simulink library "SUB_ECU_L4_MABX_HW_Interface_PIC_PB"  (R2018a)
settings: Solver=VariableStepAuto  StartTime=0.0  StopTime=10.0  RelTol=1e-3
PostLoadFcn:
  | , if any(exist('dsrtsu_mdlpostloadfcn', 'file') == [2, 3, 6]), try dsrtsu_mdlpostloadfcn('Execute', bdroot); catch fprintf('Error in PostLoadFcn (dsrtsu_mdlpostloadfcn) for model "%s":\n %s\n', bdroot, lasterr); end, end,
undefined symbols (not defined in the file or in its folder): CANR_PROPB_REAX_3_13_CHANNEL_APV, CANR_PROPB_REAX_4_13_CHANNEL_APV, CANR_PROPB_XPR_1_50_CHANNEL_APV, ENUM_CAN_RX_T, ENUM_CAN_TX_T, ENUM_REAX_OPERATION_MODE_T, ENUM_SIGNAL_HEALTH_T, ENUM_XBR_CONTROL_MODE_T, ENUM_XBR_EBI_MODE_T, ENUM_XBR_PASS_THROUGH_ACTIVE_T, ENUM_XBR_PRIORITY_T, ENUM_XPR_INHIBIT_PARK_MANUAL_T, ENUM_XPR_INHIBIT_UNPARK_MANUAL_T, ENUM_XPR_PARK_MANUAL_T, ENUM_XPR_UNPARK_MANUAL_T, PROPB_REAX_1_E4_DES_POS_SIG_SRC_APV, PROPB_REAX_1_E4_DESIRED_OPMODE_APV, PROPB_REAX_1_E4_DESIRED_POSITION_APV, PROPB_REAX_CHANNEL_APV, ptc_matlab_lib
libraries: PTC_MBDS_LIB x293, rtican x158, simulink x61, EmE_MBD_Blockset x38, rti1401lib_dio_type4 x14, simulink_need_slupdate x7, $bdroot x5, rti1401lib_adc_type4 x3, rtmapslib x3, dsa_tcpip_lib x2, SUB_ECU_L4_MABX_HW_Interface_PTC_1571 x1, rtitasklib x1
(part 3 of 49)

== system SUB_ECU_L4_MABX_HW_Interface_PIC_PB/DIGITAL ==
  ADC_TYPE4_BL1 : rti1401lib_adc_type4/ADC_TYPE4_BL1  DSProperties=struct('RTI',struct('Version',uint32(2),'BlockType',struct('isSLSource',uint8(1),'isSLSink',uint8(1),'isHWSource',uint8(0),'isHWSink',uint8(1),'isSetup',uint8(0),'isInline',uint8(1),'isNonInline',uint8(0),'isInterrupt',uint8(0),'isChannelwise',uint8(1)),'IOBoardType',{{'DS1401','STD','ADCT4'}},'UnitType','ADC','Identifier','ADC','DialogType','ML','BlockSet','NONE','SlaveProcessor','NONE'))  RTIBlockInterface=struct('InputPortsActive',0,'InputPortsWidth',int32(1),'InputPortsDataType',{{'SS_BOOLEAN'}},'InputPortsName',{{'Continue'}},'OutputPortsActive',[1 0],'OutputPortsWidth',int32([1 1]),'OutputPortsDataType',{{'SS_DOUBLE','SS_UINT8'}},'OutputPortsName',{{'ADC','Status'}},'DialogFcn','rti1401stdadct4adcgui','SampleTime',{{-1}},'InitLevel',3,'IconTransparency','on','BlockDisplay',{{['ADC TP4\nModule: 1\nChannel: 2'],'center'}},'BlockName',struct('Token',{{'ADC_TYPE4_BL1'}}))  RTIBlockParameters=struct('ADCSWStartDisable',{{0,'OFF',[0 1]}},'ModuleNo',{{1,'OFF',[1 16]}},'ChannelNo',{{2,'OFF',[1 16]}},'ConversionMode',{{1,'OFF',[1 2]}},'SampleMode',{{1,'OFF',[1 2]}},'TriggerSource',{{1,'OFF',[1 5]}},'EdgePolarity',{{1,'OFF',[1 2]}},'ConversionTriggerSource',{{2,'OFF',[1 6]}},'ConversionEdgePolarity',{{1,'OFF',[1 2]}},'ConversionPeriod',{{'1e-06','OFF',[]}},'ConversionPeriodCheck',{{0,'OFF',[]}},'BurstTriggerSource',{{1,'OFF',[1 6]}},'BurstEdgePolarity',{{1,'OFF',[1 2]}},'BurstSize',{{'10','OFF',[]}},'BurstSizeCheck',{{0,'OFF',[]}},'DataSetOffset',{{'0','OFF',[]}},'DataSetOffsetCheck',{{0,'OFF',[]}},'DataSetLength',{{'1','OFF',[]}},'DataSetLengthCheck',{{0,'OFF',[]}},'ReadMode',{{1,'OFF',[1 2]}},'SampleTime',{{'-1','OFF',[-1 inf]}},'SampleTimeCheck',{{1,'OFF',[]}},'StatusPortEnable',{{0,'OFF',[0 1]}},'VoltageRange',{{2,'OFF',[1 2]}},'TLCFileName',{{'rti1401adc_t4_adc','OFF',[]}})  RTISFcnParameters=struct('ADCSWStartDisable','int32','ModuleNo','int32','ChannelNo','int16','ConversionMode','int16','SampleMode','int16','TriggerSource','int16','EdgePolarity','int16','ConversionTriggerSource','int16','ConversionEdgePolarity','int16','ConversionPeriod','double','BurstTriggerSource','int16','BurstEdgePolarity','int16','BurstSize','int16','DataSetOffset','int16','DataSetLength','int16','ReadMode','int16','SampleTime','double','StatusPortEnable','int16','VoltageRange','int16','TLCFileName','char')  RTIBlockParaDefault=struct('ADCSWStartDisable',0,'ModuleNo',1,'ChannelNo',1,'ConversionMode',1,'SampleMode',1,'TriggerSource',1,'EdgePolarity',1,'ConversionTriggerSource',2,'ConversionEdgePolarity',1,'ConversionPeriod',1e-6,'ConversionPeriodCheck',0,'BurstTriggerSource',1,'BurstEdgePolarity',1,'BurstSize',10,'BurstSizeCheck',0,'DataSetOffset',0,'DataSetOffsetCheck',0,'DataSetLength',1,'DataSetLengthCheck',0,'ReadMode',1,'SampleTime',-1,'SampleTimeCheck',1,'StatusPortEnable',0,'VoltageRange',1,'TLCFileName','rti1401adc_t4_adc')
  ADC_TYPE4_BL2 : rti1401lib_adc_type4/ADC_TYPE4_BL1  DSProperties=struct('RTI',struct('Version',uint32(2),'BlockType',struct('isSLSource',uint8(1),'isSLSink',uint8(1),'isHWSource',uint8(0),'isHWSink',uint8(1),'isSetup',uint8(0),'isInline',uint8(1),'isNonInline',uint8(0),'isInterrupt',uint8(0),'isChannelwise',uint8(1)),'IOBoardType',{{'DS1401','STD','ADCT4'}},'UnitType','ADC','Identifier','ADC','DialogType','ML','BlockSet','NONE','SlaveProcessor','NONE'))  RTIBlockInterface=struct('InputPortsActive',0,'InputPortsWidth',int32(1),'InputPortsDataType',{{'SS_BOOLEAN'}},'InputPortsName',{{'Continue'}},'OutputPortsActive',[1 0],'OutputPortsWidth',int32([1 1]),'OutputPortsDataType',{{'SS_DOUBLE','SS_UINT8'}},'OutputPortsName',{{'ADC','Status'}},'DialogFcn','rti1401stdadct4adcgui','SampleTime',{{-1}},'InitLevel',3,'IconTransparency','on','BlockDisplay',{{['ADC TP4\nModule: 1\nChannel: 1'],'center'}},'BlockName',struct('Token',{{'ADC_TYPE4_BL1'}}))  RTIBlockParameters=struct('ADCSWStartDisable',{{0,'OFF',[0 1]}},'ModuleNo',{{1,'OFF',[1 16]}},'ChannelNo',{{1,'OFF',[1 16]}},'ConversionMode',{{1,'OFF',[1 2]}},'SampleMode',{{1,'OFF',[1 2]}},'TriggerSource',{{1,'OFF',[1 5]}},'EdgePolarity',{{1,'OFF',[1 2]}},'ConversionTriggerSource',{{2,'OFF',[1 6]}},'ConversionEdgePolarity',{{1,'OFF',[1 2]}},'ConversionPeriod',{{'1e-06','OFF',[]}},'ConversionPeriodCheck',{{0,'OFF',[]}},'BurstTriggerSource',{{1,'OFF',[1 6]}},'BurstEdgePolarity',{{1,'OFF',[1 2]}},'BurstSize',{{'10','OFF',[]}},'BurstSizeCheck',{{0,'OFF',[]}},'DataSetOffset',{{'0','OFF',[]}},'DataSetOffsetCheck',{{0,'OFF',[]}},'DataSetLength',{{'1','OFF',[]}},'DataSetLengthCheck',{{0,'OFF',[]}},'ReadMode',{{1,'OFF',[1 2]}},'SampleTime',{{'-1','OFF',[-1 inf]}},'SampleTimeCheck',{{1,'OFF',[]}},'StatusPortEnable',{{0,'OFF',[0 1]}},'VoltageRange',{{2,'OFF',[1 2]}},'TLCFileName',{{'rti1401adc_t4_adc','OFF',[]}})  RTISFcnParameters=struct('ADCSWStartDisable','int32','ModuleNo','int32','ChannelNo','int16','ConversionMode','int16','SampleMode','int16','TriggerSource','int16','EdgePolarity','int16','ConversionTriggerSource','int16','ConversionEdgePolarity','int16','ConversionPeriod','double','BurstTriggerSource','int16','BurstEdgePolarity','int16','BurstSize','int16','DataSetOffset','int16','DataSetLength','int16','ReadMode','int16','SampleTime','double','StatusPortEnable','int16','VoltageRange','int16','TLCFileName','char')  RTIBlockParaDefault=struct('ADCSWStartDisable',0,'ModuleNo',1,'ChannelNo',1,'ConversionMode',1,'SampleMode',1,'TriggerSource',1,'EdgePolarity',1,'ConversionTriggerSource',2,'ConversionEdgePolarity',1,'ConversionPeriod',1e-6,'ConversionPeriodCheck',0,'BurstTriggerSource',1,'BurstEdgePolarity',1,'BurstSize',10,'BurstSizeCheck',0,'DataSetOffset',0,'DataSetOffsetCheck',0,'DataSetLength',1,'DataSetLengthCheck',0,'ReadMode',1,'SampleTime',-1,'SampleTimeCheck',1,'StatusPortEnable',0,'VoltageRange',1,'TLCFileName','rti1401adc_t4_adc')
  ADC_TYPE4_BL3 : rti1401lib_adc_type4/ADC_TYPE4_BL1  DSProperties=struct('RTI',struct('Version',uint32(2),'BlockType',struct('isSLSource',uint8(1),'isSLSink',uint8(1),'isHWSource',uint8(0),'isHWSink',uint8(1),'isSetup',uint8(0),'isInline',uint8(1),'isNonInline',uint8(0),'isInterrupt',uint8(0),'isChannelwise',uint8(1)),'IOBoardType',{{'DS1401','STD','ADCT4'}},'UnitType','ADC','Identifier','ADC','DialogType','ML','BlockSet','NONE','SlaveProcessor','NONE'))  RTIBlockInterface=struct('InputPortsActive',0,'InputPortsWidth',int32(1),'InputPortsDataType',{{'SS_BOOLEAN'}},'InputPortsName',{{'Continue'}},'OutputPortsActive',[1 0],'OutputPortsWidth',int32([1 1]),'OutputPortsDataType',{{'SS_DOUBLE','SS_UINT8'}},'OutputPortsName',{{'ADC','Status'}},'DialogFcn','rti1401stdadct4adcgui','SampleTime',{{-1}},'InitLevel',3,'IconTransparency','on','BlockDisplay',{{['ADC TP4\nModule: 1\nChannel: 3'],'center'}},'BlockName',struct('Token',{{'ADC_TYPE4_BL1'}}))  RTIBlockParameters=struct('ADCSWStartDisable',{{0,'OFF',[0 1]}},'ModuleNo',{{1,'OFF',[1 16]}},'ChannelNo',{{3,'OFF',[1 16]}},'ConversionMode',{{1,'OFF',[1 2]}},'SampleMode',{{1,'OFF',[1 2]}},'TriggerSource',{{1,'OFF',[1 5]}},'EdgePolarity',{{1,'OFF',[1 2]}},'ConversionTriggerSource',{{2,'OFF',[1 6]}},'ConversionEdgePolarity',{{1,'OFF',[1 2]}},'ConversionPeriod',{{'1e-06','OFF',[]}},'ConversionPeriodCheck',{{0,'OFF',[]}},'BurstTriggerSource',{{1,'OFF',[1 6]}},'BurstEdgePolarity',{{1,'OFF',[1 2]}},'BurstSize',{{'10','OFF',[]}},'BurstSizeCheck',{{0,'OFF',[]}},'DataSetOffset',{{'0','OFF',[]}},'DataSetOffsetCheck',{{0,'OFF',[]}},'DataSetLength',{{'1','OFF',[]}},'DataSetLengthCheck',{{0,'OFF',[]}},'ReadMode',{{1,'OFF',[1 2]}},'SampleTime',{{'-1','OFF',[-1 inf]}},'SampleTimeCheck',{{1,'OFF',[]}},'StatusPortEnable',{{0,'OFF',[0 1]}},'VoltageRange',{{2,'OFF',[1 2]}},'TLCFileName',{{'rti1401adc_t4_adc','OFF',[]}})  RTISFcnParameters=struct('ADCSWStartDisable','int32','ModuleNo','int32','ChannelNo','int16','ConversionMode','int16','SampleMode','int16','TriggerSource','int16','EdgePolarity','int16','ConversionTriggerSource','int16','ConversionEdgePolarity','int16','ConversionPeriod','double','BurstTriggerSource','int16','BurstEdgePolarity','int16','BurstSize','int16','DataSetOffset','int16','DataSetLength','int16','ReadMode','int16','SampleTime','double','StatusPortEnable','int16','VoltageRange','int16','TLCFileName','char')  RTIBlockParaDefault=struct('ADCSWStartDisable',0,'ModuleNo',1,'ChannelNo',1,'ConversionMode',1,'SampleMode',1,'TriggerSource',1,'EdgePolarity',1,'ConversionTriggerSource',2,'ConversionEdgePolarity',1,'ConversionPeriod',1e-6,'ConversionPeriodCheck',0,'BurstTriggerSource',1,'BurstEdgePolarity',1,'BurstSize',10,'BurstSizeCheck',0,'DataSetOffset',0,'DataSetOffsetCheck',0,'DataSetLength',1,'DataSetLengthCheck',0,'ReadMode',1,'SampleTime',-1,'SampleTimeCheck',1,'StatusPortEnable',0,'VoltageRange',1,'TLCFileName','rti1401adc_t4_adc')
  Bus Creator1 : BusCreator  Inputs=13
  Constant : Constant  Value=1000
  Constant1 : Constant  Value=2000
  Constant2 : Constant  Value=1000
  Constant3 : Constant  Value=500
  DIO_TYPE4_BIT_IN_CH_1 : rti1401lib_dio_type4/DIO_TYPE4_BIT_IN_CH_BL1  DSProperties=struct('RTI',struct('Version',uint32(1),'BlockType',struct('isSLSource',uint8(1),'isSLSink',uint8(0),'isHWSource',uint8(1),'isHWSink',uint8(0),'isSetup',uint8(0),'isInline',uint8(1),'isNonInline',uint8(0),'isInterrupt',uint8(0),'isChannelwise',uint8(1)),'IOBoardType',{{'DS1401','STD','DIOT4'}},'UnitType','BIT','Identifier','BITINCH','DialogType','ML','BlockSet','NONE','SlaveProcessor','NONE'))  RTIBlockInterface=struct('OutputPortsWidth',int32(1),'OutputPortsDataType',{{'SS_BOOLEAN'}},'OutputPortsActive',1,'OutputPortsName',{{'Out'}},'BlockDisplay',{{['DIO TP4 BIT IN\n Channelwise\nModule: 1\nPort: 1\nChannel: 1'],'center'}},'IconTransparency','on','InitLevel',3,'DialogFcn','rti1401stddiot4bitinchgui','BlockName',struct('Token',{{'DIO_TYPE4_BIT_IN_CH_BL1'}}))  RTIBlockParameters=struct('ModuleNo',{{1,'OFF',[1 16]}},'PortNo',{{1,'OFF',[1 2]}},'ChannelNo',{{1,'OFF',[1 16]}},'TLCFileName',{{'rti1401dio_t4_bit_in_ch','OFF',[]}},'EnableInterrupt',{{0,'OFF',[0 1]}},'TriggerEdgeType',{{1,'OFF',[1 3]}})  RTISFcnParameters=struct('ModuleNo','int32','PortNo','int16','ChannelNo','int16','TLCFileName','char','EnableInterrupt','int16','TriggerEdgeType','int32')  RTIBlockParaDefault=struct('ModuleNo',1,'PortNo',1,'ChannelNo',1,'TLCFileName','rti1401dio_t4_bit_in_ch','EnableInterrupt',0,'TriggerEdgeType',1)
  DIO_TYPE4_BIT_IN_CH_3 : rti1401lib_dio_type4/DIO_TYPE4_BIT_IN_CH_BL1  DSProperties=struct('RTI',struct('Version',uint32(1),'BlockType',struct('isSLSource',uint8(1),'isSLSink',uint8(0),'isHWSource',uint8(1),'isHWSink',uint8(0),'isSetup',uint8(0),'isInline',uint8(1),'isNonInline',uint8(0),'isInterrupt',uint8(0),'isChannelwise',uint8(1)),'IOBoardType',{{'DS1401','STD','DIOT4'}},'UnitType','BIT','Identifier','BITINCH','DialogType','ML','BlockSet','NONE','SlaveProcessor','NONE'))  RTIBlockInterface=struct('OutputPortsWidth',int32(1),'OutputPortsDataType',{{'SS_BOOLEAN'}},'OutputPortsActive',1,'OutputPortsName',{{'Out'}},'BlockDisplay',{{['DIO TP4 BIT IN\n Channelwise\nModule: 1\nPort: 1\nChannel: 3'],'center'}},'IconTransparency','on','InitLevel',3,'DialogFcn','rti1401stddiot4bitinchgui','BlockName',struct('Token',{{'DIO_TYPE4_BIT_IN_CH_BL1'}}))  RTIBlockParameters=struct('ModuleNo',{{1,'OFF',[1 16]}},'PortNo',{{1,'OFF',[1 2]}},'ChannelNo',{{3,'OFF',[1 16]}},'TLCFileName',{{'rti1401dio_t4_bit_in_ch','OFF',[]}},'EnableInterrupt',{{0,'OFF',[0 1]}},'TriggerEdgeType',{{1,'OFF',[1 3]}})  RTISFcnParameters=struct('ModuleNo','int32','PortNo','int16','ChannelNo','int16','TLCFileName','char','EnableInterrupt','int16','TriggerEdgeType','int32')  RTIBlockParaDefault=struct('ModuleNo',1,'PortNo',1,'ChannelNo',1,'TLCFileName','rti1401dio_t4_bit_in_ch','EnableInterrupt',0,'TriggerEdgeType',1)
  DIO_TYPE4_BIT_IN_CH_4 : rti1401lib_dio_type4/DIO_TYPE4_BIT_IN_CH_BL1  DSProperties=struct('RTI',struct('Version',uint32(1),'BlockType',struct('isSLSource',uint8(1),'isSLSink',uint8(0),'isHWSource',uint8(1),'isHWSink',uint8(0),'isSetup',uint8(0),'isInline',uint8(1),'isNonInline',uint8(0),'isInterrupt',uint8(0),'isChannelwise',uint8(1)),'IOBoardType',{{'DS1401','STD','DIOT4'}},'UnitType','BIT','Identifier','BITINCH','DialogType','ML','BlockSet','NONE','SlaveProcessor','NONE'))  RTIBlockInterface=struct('OutputPortsWidth',int32(1),'OutputPortsDataType',{{'SS_BOOLEAN'}},'OutputPortsActive',1,'OutputPortsName',{{'Out'}},'BlockDisplay',{{['DIO TP4 BIT IN\n Channelwise\nModule: 1\nPort: 1\nChannel: 4'],'center'}},'IconTransparency','on','InitLevel',3,'DialogFcn','rti1401stddiot4bitinchgui','BlockName',struct('Token',{{'DIO_TYPE4_BIT_IN_CH_BL1'}}))  RTIBlockParameters=struct('ModuleNo',{{1,'OFF',[1 16]}},'PortNo',{{1,'OFF',[1 2]}},'ChannelNo',{{4,'OFF',[1 16]}},'TLCFileName',{{'rti1401dio_t4_bit_in_ch','OFF',[]}},'EnableInterrupt',{{0,'OFF',[0 1]}},'TriggerEdgeType',{{1,'OFF',[1 3]}})  RTISFcnParameters=struct('ModuleNo','int32','PortNo','int16','ChannelNo','int16','TLCFileName','char','EnableInterrupt','int16','TriggerEdgeType','int32')  RTIBlockParaDefault=struct('ModuleNo',1,'PortNo',1,'ChannelNo',1,'TLCFileName','rti1401dio_t4_bit_in_ch','EnableInterrupt',0,'TriggerEdgeType',1)
  DIO_TYPE4_BIT_IN_CH_5 : rti1401lib_dio_type4/DIO_TYPE4_BIT_IN_CH_BL1  DSProperties=struct('RTI',struct('Version',uint32(1),'BlockType',struct('isSLSource',uint8(1),'isSLSink',uint8(0),'isHWSource',uint8(1),'isHWSink',uint8(0),'isSetup',uint8(0),'isInline',uint8(1),'isNonInline',uint8(0),'isInterrupt',uint8(0),'isChannelwise',uint8(1)),'IOBoardType',{{'DS1401','STD','DIOT4'}},'UnitType','BIT','Identifier','BITINCH','DialogType','ML','BlockSet','NONE','SlaveProcessor','NONE'))  RTIBlockInterface=struct('OutputPortsWidth',int32(1),'OutputPortsDataType',{{'SS_BOOLEAN'}},'OutputPortsActive',1,'OutputPortsName',{{'Out'}},'BlockDisplay',{{['DIO TP4 BIT IN\n Channelwise\nModule: 1\nPort: 1\nChannel: 5'],'center'}},'IconTransparency','on','InitLevel',3,'DialogFcn','rti1401stddiot4bitinchgui','BlockName',struct('Token',{{'DIO_TYPE4_BIT_IN_CH_BL1'}}))  RTIBlockParameters=struct('ModuleNo',{{1,'OFF',[1 16]}},'PortNo',{{1,'OFF',[1 2]}},'ChannelNo',{{5,'OFF',[1 16]}},'TLCFileName',{{'rti1401dio_t4_bit_in_ch','OFF',[]}},'EnableInterrupt',{{0,'OFF',[0 1]}},'TriggerEdgeType',{{1,'OFF',[1 3]}})  RTISFcnParameters=struct('ModuleNo','int32','PortNo','int16','ChannelNo','int16','TLCFileName','char','EnableInterrupt','int16','TriggerEdgeType','int32')  RTIBlockParaDefault=struct('ModuleNo',1,'PortNo',1,'ChannelNo',1,'TLCFileName','rti1401dio_t4_bit_in_ch','EnableInterrupt',0,'TriggerEdgeType',1)
  DIO_TYPE4_BIT_IN_CH_6 : rti1401lib_dio_type4/DIO_TYPE4_BIT_IN_CH_BL1  DSProperties=struct('RTI',struct('Version',uint32(1),'BlockType',struct('isSLSource',uint8(1),'isSLSink',uint8(0),'isHWSource',uint8(1),'isHWSink',uint8(0),'isSetup',uint8(0),'isInline',uint8(1),'isNonInline',uint8(0),'isInterrupt',uint8(0),'isChannelwise',uint8(1)),'IOBoardType',{{'DS1401','STD','DIOT4'}},'UnitType','BIT','Identifier','BITINCH','DialogType','ML','BlockSet','NONE','SlaveProcessor','NONE'))  RTIBlockInterface=struct('OutputPortsWidth',int32(1),'OutputPortsDataType',{{'SS_BOOLEAN'}},'OutputPortsActive',1,'OutputPortsName',{{'Out'}},'BlockDisplay',{{['DIO TP4 BIT IN\n Channelwise\nModule: 1\nPort: 1\nChannel: 6'],'center'}},'IconTransparency','on','InitLevel',3,'DialogFcn','rti1401stddiot4bitinchgui','BlockName',struct('Token',{{'DIO_TYPE4_BIT_IN_CH_BL1'}}))  RTIBlockParameters=struct('ModuleNo',{{1,'OFF',[1 16]}},'PortNo',{{1,'OFF',[1 2]}},'ChannelNo',{{6,'OFF',[1 16]}},'TLCFileName',{{'rti1401dio_t4_bit_in_ch','OFF',[]}},'EnableInterrupt',{{0,'OFF',[0 1]}},'TriggerEdgeType',{{1,'OFF',[1 3]}})  RTISFcnParameters=struct('ModuleNo','int32','PortNo','int16','ChannelNo','int16','TLCFileName','char','EnableInterrupt','int16','TriggerEdgeType','int32')  RTIBlockParaDefault=struct('ModuleNo',1,'PortNo',1,'ChannelNo',1,'TLCFileName','rti1401dio_t4_bit_in_ch','EnableInterrupt',0,'TriggerEdgeType',1)
  DIO_TYPE4_BIT_IN_CH_7 : rti1401lib_dio_type4/DIO_TYPE4_BIT_IN_CH_BL1  DSProperties=struct('RTI',struct('Version',uint32(1),'BlockType',struct('isSLSource',uint8(1),'isSLSink',uint8(0),'isHWSource',uint8(1),'isHWSink',uint8(0),'isSetup',uint8(0),'isInline',uint8(1),'isNonInline',uint8(0),'isInterrupt',uint8(0),'isChannelwise',uint8(1)),'IOBoardType',{{'DS1401','STD','DIOT4'}},'UnitType','BIT','Identifier','BITINCH','DialogType','ML','BlockSet','NONE','SlaveProcessor','NONE'))  RTIBlockInterface=struct('OutputPortsWidth',int32(1),'OutputPortsDataType',{{'SS_BOOLEAN'}},'OutputPortsActive',1,'OutputPortsName',{{'Out'}},'BlockDisplay',{{['DIO TP4 BIT IN\n Channelwise\nModule: 1\nPort: 1\nChannel: 7'],'center'}},'IconTransparency','on','InitLevel',3,'DialogFcn','rti1401stddiot4bitinchgui','BlockName',struct('Token',{{'DIO_TYPE4_BIT_IN_CH_BL1'}}))  RTIBlockParameters=struct('ModuleNo',{{1,'OFF',[1 16]}},'PortNo',{{1,'OFF',[1 2]}},'ChannelNo',{{7,'OFF',[1 16]}},'TLCFileName',{{'rti1401dio_t4_bit_in_ch','OFF',[]}},'EnableInterrupt',{{0,'OFF',[0 1]}},'TriggerEdgeType',{{1,'OFF',[1 3]}})  RTISFcnParameters=struct('ModuleNo','int32','PortNo','int16','ChannelNo','int16','TLCFileName','char','EnableInterrupt','int16','TriggerEdgeType','int32')  RTIBlockParaDefault=struct('ModuleNo',1,'PortNo',1,'ChannelNo',1,'TLCFileName','rti1401dio_t4_bit_in_ch','EnableInterrupt',0,'TriggerEdgeType',1)
  DIO_TYPE4_PWM2D_BL1 : rti1401lib_dio_type4/DIO_TYPE4_PWM2D_BL1  DSProperties=struct('RTI',struct('Version',uint32(1),'BlockType',struct('isSLSource',uint8(1),'isSLSink',uint8(0),'isHWSource',uint8(1),'isHWSink',uint8(0),'isSetup',uint8(0),'isInline',uint8(1),'isNonInline',uint8(0),'isInterrupt',uint8(0),'isChannelwise',uint8(1)),'IOBoardType',{{'DS1401','STD','DIOT4'}},'UnitType','PWM','Identifier','PWM2D','DialogType','ML','BlockSet','NONE','SlaveProcessor','NONE'))  RTIBlockInterface=struct('OutputPortsWidth',int32([1 1]),'OutputPortsActive',[1 1],'OutputPortsName',{{'Frequency',['Duty Cycle']}},'BlockDisplay',{{['DIO TP4 PWM2D\nModule: 1\nPort: 1\nChannel: 2'],'center'}},'IconTransparency','on','InitLevel',3,'DialogFcn','rti1401stddiot4pwm2dgui','BlockName',struct('Token',{{'DIO_TYPE4_PWM2D_BL1'}}))  RTIBlockParameters=struct('ModuleNo',{{1,'ON',[1 16]}},'PortNo',{{1,'OFF',[1 2]}},'ChannelNo',{{2,'ON',[1 16]}},'UpdateMode',{{1,'ON',[1 2]}},'FrequencyRange',{{7,'OFF',[1 16]}},'TLCFileName',{{'rti1401dio_t4_pwm2d','OFF',[]}},'EnableInterrupt',{{0,'OFF',[0 1]}},'TriggerEdgeType',{{1,'OFF',[1 3]}})  RTISFcnParameters=struct('ModuleNo','int32','PortNo','int16','ChannelNo','int16','UpdateMode','int16','FrequencyRange','int16','TLCFileName','char','EnableInterrupt','int16','TriggerEdgeType','int32')  RTIBlockParaDefault=struct('ModuleNo',1,'PortNo',1,'ChannelNo',1,'UpdateMode',1,'FrequencyRange',7,'TLCFileName','rti1401dio_t4_pwm2d','EnableInterrupt',0,'TriggerEdgeType',1)
  DIO_TYPE4_PWM2D_BL2 : rti1401lib_dio_type4/DIO_TYPE4_PWM2D_BL1  DSProperties=struct('RTI',struct('Version',uint32(1),'BlockType',struct('isSLSource',uint8(1),'isSLSink',uint8(0),'isHWSource',uint8(1),'isHWSink',uint8(0),'isSetup',uint8(0),'isInline',uint8(1),'isNonInline',uint8(0),'isInterrupt',uint8(0),'isChannelwise',uint8(1)),'IOBoardType',{{'DS1401','STD','DIOT4'}},'UnitType','PWM','Identifier','PWM2D','DialogType','ML','BlockSet','NONE','SlaveProcessor','NONE'))  RTIBlockInterface=struct('OutputPortsWidth',int32([1 1]),'OutputPortsActive',[1 1],'OutputPortsName',{{'Frequency',['Duty Cycle']}},'BlockDisplay',{{['DIO TP4 PWM2D\nModule: 1\nPort: 2\nChannel: 1'],'center'}},'IconTransparency','on','InitLevel',3,'DialogFcn','rti1401stddiot4pwm2dgui','BlockName',struct('Token',{{'DIO_TYPE4_PWM2D_BL1'}}))  RTIBlockParameters=struct('ModuleNo',{{1,'ON',[1 16]}},'PortNo',{{2,'OFF',[1 2]}},'ChannelNo',{{1,'ON',[1 8]}},'UpdateMode',{{1,'ON',[1 2]}},'FrequencyRange',{{12,'OFF',[1 16]}},'TLCFileName',{{'rti1401dio_t4_pwm2d','OFF',[]}},'EnableInterrupt',{{0,'OFF',[0 1]}},'TriggerEdgeType',{{1,'OFF',[1 3]}})  RTISFcnParameters=struct('ModuleNo','int32','PortNo','int16','ChannelNo','int16','UpdateMode','int16','FrequencyRange','int16','TLCFileName','char','EnableInterrupt','int16','TriggerEdgeType','int32')  RTIBlockParaDefault=struct('ModuleNo',1,'PortNo',1,'ChannelNo',1,'UpdateMode',1,'FrequencyRange',7,'TLCFileName','rti1401dio_t4_pwm2d','EnableInterrupt',0,'TriggerEdgeType',1)
  DIO_TYPE4_PWM2D_BL3 : rti1401lib_dio_type4/DIO_TYPE4_PWM2D_BL1  DSProperties=struct('RTI',struct('Version',uint32(1),'BlockType',struct('isSLSource',uint8(1),'isSLSink',uint8(0),'isHWSource',uint8(1),'isHWSink',uint8(0),'isSetup',uint8(0),'isInline',uint8(1),'isNonInline',uint8(0),'isInterrupt',uint8(0),'isChannelwise',uint8(1)),'IOBoardType',{{'DS1401','STD','DIOT4'}},'UnitType','PWM','Identifier','PWM2D','DialogType','ML','BlockSet','NONE','SlaveProcessor','NONE'))  RTIBlockInterface=struct('OutputPortsWidth',int32([1 1]),'OutputPortsActive',[1 1],'OutputPortsName',{{'Frequency',['Duty Cycle']}},'BlockDisplay',{{['DIO TP4 PWM2D\nModule: 1\nPort: 2\nChannel: 2'],'center'}},'IconTransparency','on','InitLevel',3,'DialogFcn','rti1401stddiot4pwm2dgui','BlockName',struct('Token',{{'DIO_TYPE4_PWM2D_BL1'}}))  RTIBlockParameters=struct('ModuleNo',{{1,'ON',[1 16]}},'PortNo',{{2,'OFF',[1 2]}},'ChannelNo',{{2,'ON',[1 8]}},'UpdateMode',{{1,'ON',[1 2]}},'FrequencyRange',{{12,'OFF',[1 16]}},'TLCFileName',{{'rti1401dio_t4_pwm2d','OFF',[]}},'EnableInterrupt',{{0,'OFF',[0 1]}},'TriggerEdgeType',{{1,'OFF',[1 3]}})  RTISFcnParameters=struct('ModuleNo','int32','PortNo','int16','ChannelNo','int16','UpdateMode','int16','FrequencyRange','int16','TLCFileName','char','EnableInterrupt','int16','TriggerEdgeType','int32')  RTIBlockParaDefault=struct('ModuleNo',1,'PortNo',1,'ChannelNo',1,'UpdateMode',1,'FrequencyRange',7,'TLCFileName','rti1401dio_t4_pwm2d','EnableInterrupt',0,'TriggerEdgeType',1)
  Data Type Conversion{1..3,9} (4 alike) : DataTypeConversion  OutDataTypeStr=double  SaturateOnIntegerOverflow=on
  Debounce : Subsystem
  Debounce1 : $bdroot/DIGITAL/Debounce
  EStopSwActive : DataTypeConversion  OutDataTypeStr=boolean
  Gain : Gain  Gain=100
  Gain1 : Gain  Gain=100
  KL15_Monitor : Gain  Gain=10
  LogPbActive : DataTypeConversion  OutDataTypeStr=boolean
  Logical Operator{,1..3} (4 alike) : Logic  Operator=NOT  AllPortsSameDT=off  OutDataTypeStr=boolean
  PWM pedal input management : Subsystem
  ShifterControlDC : Gain
  ShifterControlDC1 : Gain
  ShifterControlDC2 : Gain
  ShifterControlFreq : Gain
  Signal Check : Subsystem
  StartPBActive : DataTypeConversion  OutDataTypeStr=boolean
  StartPBActive1 : DataTypeConversion  OutDataTypeStr=boolean
  Terminator : Terminator
  Terminator1 : Terminator
  DIO_bus : Outport
  wires:
  EStopSwActive/1 -> Logical Operator1/1
  DIO_TYPE4_BIT_IN_CH_4/1 -> Signal Check/2(NC)  "EnableSW_NC"
  DIO_TYPE4_PWM2D_BL2/2 -> Gain/1
  KL15_Monitor/1 -> Bus Creator1/13  "IgnitionKeySwitch_voltage"
  DIO_TYPE4_PWM2D_BL2/1 -> Data Type Conversion2/1
  DIO_TYPE4_BIT_IN_CH_3/1 -> EStopSwActive/1
  ADC_TYPE4_BL3/1 -> KL15_Monitor/1
  DIO_TYPE4_PWM2D_BL1/2 -> ShifterControlDC/1
  PWM pedal input management/1(Pedal_pwm_position) -> Bus Creator1/12  "Pedal_pwm_position"
  ShifterControlDC2/1 -> Terminator1/1
  ShifterControlDC1/1 -> Terminator/1
  Bus Creator1/1 -> DIO_bus/1
  ADC_TYPE4_BL1/1 -> ShifterControlDC2/1
  DIO_TYPE4_PWM2D_BL3/2 -> Gain1/1
  ADC_TYPE4_BL2/1 -> ShifterControlDC1/1
  DIO_TYPE4_PWM2D_BL3/1 -> Data Type Conversion3/1
  ShifterControlDC/1 -> Bus Creator1/7  "ShiftControlDC"
  Data Type Conversion2/1 -> Bus Creator1/8, PWM pedal input management/1(Pedal_1_pwm_freq_raw_value)  "Pedal_1_pwm_freq_raw_value"
  Gain/1 -> Data Type Conversion9/1
  Gain1/1 -> Data Type Conversion1/1
  ShifterControlFreq/1 -> Bus Creator1/6  "ShiftControlFreq"
  Data Type Conversion1/1 -> PWM pedal input management/4(Pedal_2_pwm_dc_raw_value), Bus Creator1/11  "Pedal_2_pwm_dc_raw_value"
  DIO_TYPE4_BIT_IN_CH_1/1 -> Signal Check/1(NO)  "EnableSW_NO"
  Data Type Conversion9/1 -> PWM pedal input management/2(Pedal_1_pwm_dc_raw_value), Bus Creator1/9  "Pedal_1_pwm_dc_raw_value"
  DIO_TYPE4_PWM2D_BL1/1 -> ShifterControlFreq/1
  Data Type Conversion3/1 -> PWM pedal input management/3(Pedal_2_pwm_freq_raw_value), Bus Creator1/10  "Pedal_2_pwm_freq_raw_value"
  DIO_TYPE4_BIT_IN_CH_5/1 -> StartPBActive/1
  Debounce1/1 -> Bus Creator1/2  "EngagePB"
  Signal Check/1(Out) -> Bus Creator1/1  "EnableSw"
  StartPBActive/1 -> Logical Operator/1
  Logical Operator1/1 -> Bus Creator1/3  "EStop"
  DIO_TYPE4_BIT_IN_CH_6/1 -> LogPbActive/1
  LogPbActive/1 -> Logical Operator2/1
  Debounce/1(Out) -> Bus Creator1/4  "LogEventPB"
  Constant1/1 -> Debounce/3(Off_Delay_ms)
  Constant/1 -> Debounce/2(On_Delay_ms)
  Logical Operator2/1 -> Debounce/1(In)
  Logical Operator3/1 -> Bus Creator1/5  "BrakeSW"
  StartPBActive1/1 -> Logical Operator3/1
  DIO_TYPE4_BIT_IN_CH_7/1 -> StartPBActive1/1
  Logical Operator/1 -> Debounce1/1
  Constant2/1 -> Debounce1/2
  Constant3/1 -> Debounce1/3

== system SUB_ECU_L4_MABX_HW_Interface_PIC_PB/DIGITAL_out ==
  Out : Inport
  In : Inport  Port=2
  Bus Selector : BusSelector  OutputSignals=10msTask.APTC.APTC_arb_pedal_position,10msTask.AutonomousState.AutonomousOutputEnabled
  Constant1 : Constant
  Constant2 : Constant  Value=0.001
  Constant3 : Constant
  Constant4 : Constant  Value=0.001
  DIO_TYPE4_BIT_OUT_CH_BL1 : rti1401lib_dio_type4/DIO_TYPE4_BIT_OUT_CH_BL1  DSProperties=struct('RTI',struct('Version',uint32(1),'BlockType',struct('isSLSource',uint8(0),'isSLSink',uint8(1),'isHWSource',uint8(0),'isHWSink',uint8(1),'isSetup',uint8(0),'isInline',uint8(1),'isNonInline',uint8(0),'isInterrupt',uint8(0),'isChannelwise',uint8(1)),'IOBoardType',{{'DS1401','STD','DIOT4'}},'UnitType','BIT','Identifier','BITOUTCH','DialogType','ML','BlockSet','NONE','SlaveProcessor','NONE'))  RTIBlockInterface=struct('InputPortsWidth',int32(1),'InputPortsActive',1,'InputPortsDataType',{{'SS_BOOLEAN'}},'InputPortsName',{{'In'}},'BlockDisplay',{{['DIO TP4 BIT OUT\n Channelwise\nModule: 1\nPort: 1\nChannel: 1'],'center'}},'IconTransparency','on','InitLevel',3,'DialogFcn','rti1401stddiot4bitoutchgui','BlockName',struct('Token',{{'DIO_TYPE4_BIT_OUT_CH_BL1'}}))  RTIBlockParameters=struct('ModuleNo',{{1,'OFF',[1 16]}},'PortNo',{{1,'OFF',[1 2]}},'ChannelNo',{{1,'OFF',[1 16]}},'OutputStateInit',{{0,'OFF',[0 1]}},'TerminationMode',{{0,'OFF',[0 1]}},'OutputStateTermValidate',{{0,'OFF',[0 1]}},'OutputStateTerm',{{0,'OFF',[0 1]}},'SupplyRailsCh',{{[0 1],'OFF',[0 1 0 1]}},'TLCFileName',{{'rti1401dio_t4_bit_out_ch','OFF',[]}},'EnableInterrupt',{{0,'OFF',[0 1]}},'TriggerEdgeType',{{1,'OFF',[1 3]}})  RTISFcnParameters=struct('ModuleNo','int32','PortNo','int16','ChannelNo','int16','SupplyRailsCh','int16','OutputStateInit','int16','TerminationMode','int16','OutputStateTermValidate','int16','OutputStateTerm','int16','TLCFileName','char','EnableInterrupt','int16','TriggerEdgeType','int32')  RTIBlockParaDefault=struct('ModuleNo',1,'PortNo',1,'ChannelNo',1,'OutputStateInit',0,'TerminationMode',0,'OutputStateTermValidate',0,'OutputStateTerm',0,'SupplyRailsCh',[1 1],'TLCFileName','rti1401dio_t4_bit_out_ch','EnableInterrupt',0,'TriggerEdgeType',1)
  DIO_TYPE4_BIT_OUT_CH_BL2 : rti1401lib_dio_type4/DIO_TYPE4_BIT_OUT_CH_BL1  DSProperties=struct('RTI',struct('Version',uint32(1),'BlockType',struct('isSLSource',uint8(0),'isSLSink',uint8(1),'isHWSource',uint8(0),'isHWSink',uint8(1),'isSetup',uint8(0),'isInline',uint8(1),'isNonInline',uint8(0),'isInterrupt',uint8(0),'isChannelwise',uint8(1)),'IOBoardType',{{'DS1401','STD','DIOT4'}},'UnitType','BIT','Identifier','BITOUTCH','DialogType','ML','BlockSet','NONE','SlaveProcessor','NONE'))  RTIBlockInterface=struct('InputPortsWidth',int32(1),'InputPortsActive',1,'InputPortsDataType',{{'SS_BOOLEAN'}},'InputPortsName',{{'In'}},'BlockDisplay',{{['DIO TP4 BIT OUT\n Channelwise\nModule: 1\nPort: 1\nChannel: 2'],'center'}},'IconTransparency','on','InitLevel',3,'DialogFcn','rti1401stddiot4bitoutchgui','BlockName',struct('Token',{{'DIO_TYPE4_BIT_OUT_CH_BL1'}}))  RTIBlockParameters=struct('ModuleNo',{{1,'OFF',[1 16]}},'PortNo',{{1,'OFF',[1 2]}},'ChannelNo',{{2,'OFF',[1 16]}},'OutputStateInit',{{0,'OFF',[0 1]}},'TerminationMode',{{0,'OFF',[0 1]}},'OutputStateTermValidate',{{0,'OFF',[0 1]}},'OutputStateTerm',{{0,'OFF',[0 1]}},'SupplyRailsCh',{{[0 1],'OFF',[0 1 0 1]}},'TLCFileName',{{'rti1401dio_t4_bit_out_ch','OFF',[]}},'EnableInterrupt',{{0,'OFF',[0 1]}},'TriggerEdgeType',{{1,'OFF',[1 3]}})  RTISFcnParameters=struct('ModuleNo','int32','PortNo','int16','ChannelNo','int16','SupplyRailsCh','int16','OutputStateInit','int16','TerminationMode','int16','OutputStateTermValidate','int16','OutputStateTerm','int16','TLCFileName','char','EnableInterrupt','int16','TriggerEdgeType','int32')  RTIBlockParaDefault=struct('ModuleNo',1,'PortNo',1,'ChannelNo',1,'OutputStateInit',0,'TerminationMode',0,'OutputStateTermValidate',0,'OutputStateTerm',0,'SupplyRailsCh',[1 1],'TLCFileName','rti1401dio_t4_bit_out_ch','EnableInterrupt',0,'TriggerEdgeType',1)
  DIO_TYPE4_BIT_OUT_CH_BL6 : rti1401lib_dio_type4/DIO_TYPE4_BIT_OUT_CH_BL1  DSProperties=struct('RTI',struct('Version',uint32(1),'BlockType',struct('isSLSource',uint8(0),'isSLSink',uint8(1),'isHWSource',uint8(0),'isHWSink',uint8(1),'isSetup',uint8(0),'isInline',uint8(1),'isNonInline',uint8(0),'isInterrupt',uint8(0),'isChannelwise',uint8(1)),'IOBoardType',{{'DS1401','STD','DIOT4'}},'UnitType','BIT','Identifier','BITOUTCH','DialogType','ML','BlockSet','NONE','SlaveProcessor','NONE'))  RTIBlockInterface=struct('InputPortsWidth',int32(1),'InputPortsActive',1,'InputPortsDataType',{{'SS_BOOLEAN'}},'InputPortsName',{{'In'}},'BlockDisplay',{{['DIO TP4 BIT OUT\n Channelwise\nModule: 1\nPort: 2\nChannel: 6'],'center'}},'IconTransparency','on','InitLevel',3,'DialogFcn','rti1401stddiot4bitoutchgui','BlockName',struct('Token',{{'DIO_TYPE4_BIT_OUT_CH_BL1'}}))  RTIBlockParameters=struct('ModuleNo',{{1,'OFF',[1 16]}},'PortNo',{{2,'OFF',[1 2]}},'ChannelNo',{{6,'OFF',[1 8]}},'OutputStateInit',{{0,'OFF',[0 1]}},'TerminationMode',{{0,'OFF',[0 1]}},'OutputStateTermValidate',{{0,'OFF',[0 1]}},'OutputStateTerm',{{0,'OFF',[0 1]}},'SupplyRailsCh',{{[0 1],'OFF',[0 1 0 1]}},'TLCFileName',{{'rti1401dio_t4_bit_out_ch','OFF',[]}},'EnableInterrupt',{{0,'OFF',[0 1]}},'TriggerEdgeType',{{1,'OFF',[1 3]}})  RTISFcnParameters=struct('ModuleNo','int32','PortNo','int16','ChannelNo','int16','SupplyRailsCh','int16','OutputStateInit','int16','TerminationMode','int16','OutputStateTermValidate','int16','OutputStateTerm','int16','TLCFileName','char','EnableInterrupt','int16','TriggerEdgeType','int32')  RTIBlockParaDefault=struct('ModuleNo',1,'PortNo',1,'ChannelNo',1,'OutputStateInit',0,'TerminationMode',0,'OutputStateTermValidate',0,'OutputStateTerm',0,'SupplyRailsCh',[1 1],'TLCFileName','rti1401dio_t4_bit_out_ch','EnableInterrupt',0,'TriggerEdgeType',1)
  DIO_TYPE4_PWM_BL1 : rti1401lib_dio_type4/DIO_TYPE4_PWM_BL1  DSProperties=struct('RTI',struct('Version',uint32(1),'BlockType',struct('isSLSource',uint8(0),'isSLSink',uint8(1),'isHWSource',uint8(0),'isHWSink',uint8(1),'isSetup',uint8(0),'isInline',uint8(1),'isNonInline',uint8(0),'isInterrupt',uint8(0),'isChannelwise',uint8(1)),'IOBoardType',{{'DS1401','STD','DIOT4'}},'UnitType','PWM','Identifier','PWM','DialogType','ML','BlockSet','NONE','SlaveProcessor','NONE'))  RTIBlockInterface=struct('InputPortsWidth',int32([1 1]),'InputPortsActive',[1 1],'InputPortsName',{{'Period',['Duty Cycle']}},'BlockDisplay',{{['DIO TP4 PWM\nModule: 1\nPort: 2\nChannel: 1'],'center'}},'IconTransparency','on','InitLevel',3,'DialogFcn','rti1401stddiot4pwmgui','BlockName',struct('Token',{{'DIO_TYPE4_PWM_BL1'}}))  RTIBlockParameters=struct('ModuleNo',{{1,'OFF',[1 16]}},'PortNo',{{2,'OFF',[1 2]}},'ChannelNo',{{1,'OFF',[1 8]}},'SupplyRailsCh',{{[1 0],'OFF',[0 1 0 1]}},'UpdateMode',{{1,'ON',[1 2]}},'PeriodRange',{{2,'OFF',[1 16]}},'DutyCycleInit',{{'0.1','OFF',[0 1]}},'PeriodInit',{{'5e-03','OFF',[]}},'TerminationMode',{{0,'OFF',[0 1]}},'OutputTermValidate',{{0,'OFF',[0 1]}},'OutputTermBuildCheck',{{0,'OFF',[]}},'DutyCycleTerm',{{'0','OFF',[0 1]}},'PeriodTerm',{{'5e-05','OFF',[]}},'TLCFileName',{{'rti1401dio_t4_pwm','OFF',[]}},'EnableInterrupt',{{0,'OFF',[0 1]}},'TriggerEdgeType',{{1,'OFF',[1 3]}})  RTISFcnParameters=struct('ModuleNo','int32','PortNo','int16','ChannelNo','int16','SupplyRailsCh','int16','UpdateMode','int16','PeriodRange','int16','DutyCycleInit','double','PeriodInit','double','TerminationMode','int16','OutputTermValidate','int16','DutyCycleTerm','double','PeriodTerm','double','TLCFileName','char','EnableInterrupt','int16','TriggerEdgeType','int32')  RTIBlockParaDefault=struct('ModuleNo',1,'PortNo',1,'ChannelNo',1,'SupplyRailsCh',[1 1],'UpdateMode',1,'PeriodRange',7,'DutyCycleInit',0,'PeriodInit',5e-5,'TerminationMode',0,'OutputTermValidate',0,'OutputTermBuildCheck',0,'DutyCycleTerm',0,'PeriodTerm',5e-5,'TLCFileName','rti1401dio_t4_pwm','EnableInterrupt',0,'TriggerEdgeType',1)
  DIO_TYPE4_PWM_BL2 : rti1401lib_dio_type4/DIO_TYPE4_PWM_BL1  DSProperties=struct('RTI',struct('Version',uint32(1),'BlockType',struct('isSLSource',uint8(0),'isSLSink',uint8(1),'isHWSource',uint8(0),'isHWSink',uint8(1),'isSetup',uint8(0),'isInline',uint8(1),'isNonInline',uint8(0),'isInterrupt',uint8(0),'isChannelwise',uint8(1)),'IOBoardType',{{'DS1401','STD','DIOT4'}},'UnitType','PWM','Identifier','PWM','DialogType','ML','BlockSet','NONE','SlaveProcessor','NONE'))  RTIBlockInterface=struct('InputPortsWidth',int32([1 1]),'InputPortsActive',[1 1],'InputPortsName',{{'Period',['Duty Cycle']}},'BlockDisplay',{{['DIO TP4 PWM\nModule: 1\nPort: 2\nChannel: 2'],'center'}},'IconTransparency','on','InitLevel',3,'DialogFcn','rti1401stddiot4pwmgui','BlockName',struct('Token',{{'DIO_TYPE4_PWM_BL1'}}))  RTIBlockParameters=struct('ModuleNo',{{1,'OFF',[1 16]}},'PortNo',{{2,'OFF',[1 2]}},'ChannelNo',{{2,'OFF',[1 8]}},'SupplyRailsCh',{{[1 0],'OFF',[0 1 0 1]}},'UpdateMode',{{1,'ON',[1 2]}},'PeriodRange',{{2,'OFF',[1 16]}},'DutyCycleInit',{{'0.2','OFF',[0 1]}},'PeriodInit',{{'5e-03','OFF',[]}},'TerminationMode',{{0,'OFF',[0 1]}},'OutputTermValidate',{{0,'OFF',[0 1]}},'OutputTermBuildCheck',{{0,'OFF',[]}},'DutyCycleTerm',{{'0','OFF',[0 1]}},'PeriodTerm',{{'5e-05','OFF',[]}},'TLCFileName',{{'rti1401dio_t4_pwm','OFF',[]}},'EnableInterrupt',{{0,'OFF',[0 1]}},'TriggerEdgeType',{{1,'OFF',[1 3]}})  RTISFcnParameters=struct('ModuleNo','int32','PortNo','int16','ChannelNo','int16','SupplyRailsCh','int16','UpdateMode','int16','PeriodRange','int16','DutyCycleInit','double','PeriodInit','double','TerminationMode','int16','OutputTermValidate','int16','DutyCycleTerm','double','PeriodTerm','double','TLCFileName','char','EnableInterrupt','int16','TriggerEdgeType','int32')  RTIBlockParaDefault=struct('ModuleNo',1,'PortNo',1,'ChannelNo',1,'SupplyRailsCh',[1 1],'UpdateMode',1,'PeriodRange',7,'DutyCycleInit',0,'PeriodInit',5e-5,'TerminationMode',0,'OutputTermValidate',0,'OutputTermBuildCheck',0,'DutyCycleTerm',0,'PeriodTerm',5e-5,'TLCFileName','rti1401dio_t4_pwm','EnableInterrupt',0,'TriggerEdgeType',1)
  Data Type Conversion{1..2,5..6,9..10} (6 alike) : DataTypeConversion  OutDataTypeStr=double
  Determine pedal PWM and duty cycle values : Subsystem
  Divide : Product  Inputs=*/
  Divide1 : Product  Inputs=*/
  Gain : Gain  Gain=0.01
  Gain1 : Gain  Gain=0.01
  Logical Operator : Logic  Operator=NOT  AllPortsSameDT=off  OutDataTypeStr=boolean
  MinMax : MinMax  Function=max  Inputs=2  InputSameDT=on
  MinMax1 : MinMax  Function=max  Inputs=2  InputSameDT=on
  Shift Control : Subsystem
  Status Indicator Lights : Subsystem
  Terminator : Terminator
  wires:
  Bus Selector/2 -> Determine pedal PWM and duty cycle values/2(AutonomousEnabled)  "<AutonomousOutputEnabled>"
  Status Indicator Lights/3(Red) -> DIO_TYPE4_BIT_OUT_CH_BL6/1  "RedLED"
  Determine pedal PWM and duty cycle values/3(APTC_PWM_pedalB_freq_out) -> MinMax1/1
  Determine pedal PWM and duty cycle values/1(APTC_PWM_pedalA_freq_out) -> MinMax/1
  MinMax/1 -> Data Type Conversion1/1
  MinMax1/1 -> Data Type Conversion2/1
  Constant4/1 -> MinMax1/2
  Constant2/1 -> MinMax/2
  Data Type Conversion10/1 -> DIO_TYPE4_PWM_BL2/2  "PWMOut_P2C2_DC"
  Data Type Conversion9/1 -> DIO_TYPE4_PWM_BL2/1  "PWMOut_P2C2_Period"
  Data Type Conversion6/1 -> DIO_TYPE4_PWM_BL1/2  "PWMOut_P2C1_DC"
  Data Type Conversion5/1 -> DIO_TYPE4_PWM_BL1/1  "PWMOut_P2C1_Period"
  Data Type Conversion2/1 -> Divide1/2
  Data Type Conversion1/1 -> Divide/2
  Gain1/1 -> Data Type Conversion6/1
  Gain/1 -> Data Type Conversion10/1
  Divide1/1 -> Data Type Conversion9/1
  Constant1/1 -> Divide1/1
  Divide/1 -> Data Type Conversion5/1
  Constant3/1 -> Divide/1
  Determine pedal PWM and duty cycle values/4(APTC_PWM_pedalB_DC_out) -> Gain/1
  Determine pedal PWM and duty cycle values/2(APTC_PWM_pedalA_DC_out) -> Gain1/1
  Out/1 -> Status Indicator Lights/1(Outputs), Bus Selector/1
  Shift Control/1(Out) -> Logical Operator/1
  Logical Operator/1 -> Terminator/1
  In/1 -> Determine pedal PWM and duty cycle values/3(In), Shift Control/1(In)
  Bus Selector/1 -> Determine pedal PWM and duty cycle values/1(APTC_arb_pedal_position)  "<APTC_arb_pedal_position>"
  Status Indicator Lights/1(Blue) -> DIO_TYPE4_BIT_OUT_CH_BL1/1  "BlueLED"
  Status Indicator Lights/2(Green) -> DIO_TYPE4_BIT_OUT_CH_BL2/1  "GreenLED"

== system SUB_ECU_L4_MABX_HW_Interface_PIC_PB/ETHERNET ==
  Outputs : Inport
  Data RX : Subsystem
  Data TX : Subsystem
  Enable : Constant  OutDataTypeStr=boolean
  TCPIP_Setup : dsa_tcpip_lib/TCPIP_Setup  boardType=ETH Type 1  boardNo=1  channelNo=1  localIpAddr=10.120.128.20/23
      link override Interrupt_Task/Tcp Input Processing: TriggerPort=function-call  EnablePort=none  ThBlk=struct('blkh',118342.00012207031,'srcId','SWI1','srcSgnId','SWI1','intervalTmrBlockId',[],'srcSgnName',['Software Trigger'],'srcCpuId','','isSrcCpu',1,'isTargetCpu',1,'srcOnMasterCpu',1,'boardType','','boardTypeNo','','boardNo',1,'intNo',0,'subIntNo',-1,'period',0,'entryPoint','rti_SWI1','blockName',['Tcp Input Processing'],'taskNameDisplayExt','','taskType','SWINT','groupId','SWINT','hookFcn','NULL','isTimerTaskSrc',0,'service','','mpBlkId','','taskPriorityPreConfig','none','taskPriority',-1,'taskSortWeighting',[],'taskSchedulingPolicy','FCFS','taskOvrPreConfig','none','taskOvrStrategy',1,'taskOvrQueueSize',1,'taskVisibility','on','taskGroupId','','taskGroupDisplayOrder',[],'serviceDynamicGen',0,'disableCodeGen',0,'boardBase','0','noBoardBase','')  TLCFileName=rti_swinterrupt
      settings: SourceProductName=dSPACE MABX TCP/IP Blockset
  UDPIP_Communication : dsa_tcpip_lib/UDPIP_Communication  localPort=50000  remoteAddrStr=10.120.128.10  remotePort=50000  inputSize=24  outputSize=128  legacyMode=off
      settings: SourceProductName=dSPACE MABX TCP/IP Blockset
  Unit_Delay : UnitDelay  SampleTime=-1
      settings: AttributesFormatString=IC: %<vinit>
  Update_RTMaps_Interface : rtmapslib/Update_RTMaps_Interface  SystemSampleTime=-1
      settings: SourceProductName=dSPACE RTMaps Interface Blockset
  PIC_Bus : Outport
  wires:
  Unit_Delay/1 -> Data TX/1(In)
  UDPIP_Communication/3 -> Data RX/4(DataReceived)
  Enable/1 -> UDPIP_Communication/1
  Data RX/1(PIC_Bus) -> PIC_Bus/1  "PIC_Bus"
  TCPIP_Setup/1 -> Data RX/1(LinkStatus)  "EthernetLinkStatus"
  UDPIP_Communication/1 -> Data RX/2(Status)
  Data TX/2(DataToSend) -> UDPIP_Communication/3
  Data TX/1(SizeToSend) -> UDPIP_Communication/2
  Outputs/1 -> Unit_Delay/1
  UDPIP_Communication/2 -> Data RX/3(SizeReceived)  "size_uint32"

== system SUB_ECU_L4_MABX_HW_Interface_PIC_PB/INPUTS_PIC_PB ==
  PIC_Bus : Inport
  Bus Creator : BusCreator  Inputs=4
  CAN_PIC_PB : Subsystem
  DIGITAL : $bdroot/DIGITAL
  Timer_Access : Subsystem
  Inputs : Outport
  wires:
  PIC_Bus/1 -> Bus Creator/3
  CAN_PIC_PB/1(CAN_RX) -> Bus Creator/1  "CAN"
  Bus Creator/1 -> Inputs/1  "INPUTS"
  DIGITAL/1 -> Bus Creator/2  "DIO_Bus"
  Timer_Access/1(TimeStamp) -> CAN_PIC_PB/1(timeStamp), Bus Creator/4  "timeStamp"

== system SUB_ECU_L4_MABX_HW_Interface_PIC_PB/OUTPUTS_PIC_PB ==
  Outputs : Inport
  In : Inport  Port=2
  CAN_Out_PIC_PB : Subsystem
  DIGITAL_out : $bdroot/DIGITAL_out
  wires:
  Outputs/1 -> DIGITAL_out/1, CAN_Out_PIC_PB/1(Out)
  In/1 -> DIGITAL_out/2, CAN_Out_PIC_PB/2(In)

== system SUB_ECU_L4_MABX_HW_Interface_PIC_PB/CAN_Out_PIC_PB/CAN_TX_10000ms ==
  10000msCAN : Inport
  Terminator : Terminator
  wires:
  10000msCAN/1 -> Terminator/1

== system SUB_ECU_L4_MABX_HW_Interface_PIC_PB/CAN_Out_PIC_PB/CAN_TX_1000ms ==
  1000msCAN : Inport
  CAN_TX_AIR1_31 : Subsystem
  CAN_TX_AMB_00 : Subsystem
  Constant1 : Constant  Value=ENUM_CAN_TX_T.TX_CAN_4
  Constant2 : Constant  Value=ENUM_CAN_TX_T.TX_CAN_4
  wires:
  Constant1/1 -> CAN_TX_AMB_00/1(Channel)
  1000msCAN/1 -> CAN_TX_AIR1_31/2(Data), CAN_TX_AMB_00/2(Data)
  Constant2/1 -> CAN_TX_AIR1_31/1(Channel)

== system SUB_ECU_L4_MABX_HW_Interface_PIC_PB/CAN_Out_PIC_PB/CAN_TX_100ms ==
  100msCAN : Inport
  Feedthrough : Inport  Port=2
  Bus Selector1 : BusSelector  OutputSignals=INPUTS.DIO_Bus.OperatorEnableSwitch
  Bus Selector2 : BusSelector  OutputSignals=INPUTS.DIO_Bus.OperatorEnableSwitch
  CANT_PROPB_XPR_FC_CHANNEL_APV : Constant  Value=ENUM_CAN_TX_T.TX_CAN_4
  CAN_TX_CCVS1_00 : Subsystem
  CAN_TX_PROPB_REAX_5_E4 : Subsystem
  CAN_TX_PROPB_XPR_FC : Subsystem
  COGSRapidUpdate : Subsystem
  EBC1_8B : Subsystem
  EffortsValue : Subsystem
  Encode_PropB_REAX_5 : Subsystem
  Encode_PropB_XPR_FC : Subsystem  SystemSampleTime=0.1
  POSRapidUpdate : Subsystem
  PROPB_XPR_INHIBIT_PARK_MANUAL_APV : Constant  Value=ENUM_XPR_INHIBIT_PARK_MANUAL_T.NO_OVERRIDE
  PROPB_XPR_INHIBIT_UNPARK_MANUAL_APV : Constant  Value=ENUM_XPR_INHIBIT_UNPARK_MANUAL_T.NO_OVERRIDE
  PROPB_XPR_PARK_MANUAL_APV : Constant  Value=ENUM_XPR_PARK_MANUAL_T.NO_OVERRIDE
  PROPB_XPR_UNPARK_MANUAL_APV : Constant  Value=ENUM_XPR_UNPARK_MANUAL_T.NO_OVERRIDE
  enableCOGSRapidUpdateTX : Constant  Value=boolean(1)
  enableEBC1_8B_TX : Constant  Value=boolean(1)
  enablePosRapidUpdateTX : Constant  Value=boolean(1)
  wires:
  Feedthrough/1 -> CAN_TX_CCVS1_00/1(Data), CAN_TX_PROPB_REAX_5_E4/1(enable), EBC1_8B/2(Data), COGSRapidUpdate/2(Data)
  Bus Selector2/1 -> CAN_TX_PROPB_XPR_FC/1(Enable)  "<OperatorEnableSwitch>"
  enableEBC1_8B_TX/1 -> EBC1_8B/1(Enable)
  Encode_PropB_REAX_5/1(Data) -> CAN_TX_PROPB_REAX_5_E4/2(RawData)
  EffortsValue/1(EffortsValue) -> Encode_PropB_REAX_5/1(EffortsValue)
  Bus Selector1/1 -> Encode_PropB_XPR_FC/5(F_MessageEnable)  "<OperatorEnableSwitch>"
  CANT_PROPB_XPR_FC_CHANNEL_APV/1 -> CAN_TX_PROPB_XPR_FC/2(Channel)
  Encode_PropB_XPR_FC/1(Data) -> CAN_TX_PROPB_XPR_FC/3(RawData)
  PROPB_XPR_INHIBIT_UNPARK_MANUAL_APV/1 -> Encode_PropB_XPR_FC/2(inhibit_unpark_manual)
  PROPB_XPR_PARK_MANUAL_APV/1 -> Encode_PropB_XPR_FC/3(park_manual)
  PROPB_XPR_UNPARK_MANUAL_APV/1 -> Encode_PropB_XPR_FC/4(unpark_manual)
  PROPB_XPR_INHIBIT_PARK_MANUAL_APV/1 -> Encode_PropB_XPR_FC/1(inhibit_park_manual)
  enableCOGSRapidUpdateTX/1 -> COGSRapidUpdate/1(Enable)
  enablePosRapidUpdateTX/1 -> POSRapidUpdate/1(Enable)
  100msCAN/1 -> Bus Selector2/1, Bus Selector1/1, POSRapidUpdate/2(Data)

== system SUB_ECU_L4_MABX_HW_Interface_PIC_PB/CAN_Out_PIC_PB/CAN_TX_10ms ==
  10msCAN : Inport
  In : Inport  Port=2
  CANT_ACCS_E4_CHANNEL_APV : Constant  Value=ENUM_CAN_TX_T.TX_CAN_4
  CANT_EEC1_00_CHANNEL_APV : Constant  Value=ENUM_CAN_TX_T.TX_CAN_4_5
  CANT_VDC2_0B_CHANNEL_APV : Constant  Value=ENUM_CAN_TX_T.TX_CAN_5
  CAN_TX_ACCS_E4 : Subsystem
  CAN_TX_EEC1_00 : Subsystem
  CAN_TX_PROPB_REAX_1_E4 : Subsystem
  CAN_TX_VDC2_0B : Subsystem
  Encode_PROPB_REAX_1 : Subsystem
  wires:
  In/1 -> CAN_TX_EEC1_00/2(Data), CAN_TX_PROPB_REAX_1_E4/1(enable)
  CANT_ACCS_E4_CHANNEL_APV/1 -> CAN_TX_ACCS_E4/1(Channel)
  CANT_EEC1_00_CHANNEL_APV/1 -> CAN_TX_EEC1_00/1(Channel)
  Encode_PROPB_REAX_1/1(Out1) -> CAN_TX_PROPB_REAX_1_E4/2(RawData)
  CANT_VDC2_0B_CHANNEL_APV/1 -> CAN_TX_VDC2_0B/1(Channel)
  10msCAN/1 -> CAN_TX_VDC2_0B/2(Data), CAN_TX_ACCS_E4/2(Data), Encode_PROPB_REAX_1/1(In1)

== system SUB_ECU_L4_MABX_HW_Interface_PIC_PB/CAN_Out_PIC_PB/CAN_TX_20ms ==
  20msCAN : Inport
  Bus Selector : BusSelector  OutputSignals=INPUTS.DIO_Bus.OperatorEnableSwitch
  CANT_PROPB_XBR_B3_CHANNEL_APV : Constant  Value=0
  CANT_STD_ODOMETRY_CHANNEL_APV : Constant  Value=ENUM_CAN_TX_T.TX_CAN_6
  CAN_TX_PROPB_XBR_B3 : Subsystem
  CAN_TX_PropB_2C2_XPR_65 : Subsystem
  CAN_TX_STD_ODOMETRY : Subsystem
  Encode_PropB_2C2_XPR : Subsystem
  Encode_PropB_XBR_B3 : Subsystem
  wires:
  20msCAN/1 -> CAN_TX_STD_ODOMETRY/2(Data), Encode_PropB_XBR_B3/1(In), Bus Selector/1, Encode_PropB_2C2_XPR/1(In)
  Encode_PropB_2C2_XPR/1(F_2C2_Enable) -> CAN_TX_PropB_2C2_XPR_65/1(Enable)
  Encode_PropB_2C2_XPR/2(Out) -> CAN_TX_PropB_2C2_XPR_65/2(RawData)
  Bus Selector/1 -> CAN_TX_PROPB_XBR_B3/3(OperatorEnable)  "<OperatorEnableSwitch>"
  Encode_PropB_XBR_B3/1(Out) -> CAN_TX_PROPB_XBR_B3/2(Data)
  CANT_PROPB_XBR_B3_CHANNEL_APV/1 -> CAN_TX_PROPB_XBR_B3/1(Channel)
  CANT_STD_ODOMETRY_CHANNEL_APV/1 -> CAN_TX_STD_ODOMETRY/1(Channel)

== system SUB_ECU_L4_MABX_HW_Interface_PIC_PB/CAN_Out_PIC_PB/CAN_TX_250ms ==
  250msCAN : Inport
  Terminator : Terminator
  wires:
  250msCAN/1 -> Terminator/1

== system SUB_ECU_L4_MABX_HW_Interface_PIC_PB/CAN_Out_PIC_PB/CAN_TX_5000ms ==
  5000msCAN : Inport
  Bus Selector : BusSelector  OutputSignals=INPUTS.DIO_Bus.OperatorEnableSwitch
  CAN_TX_RQST_13_E4 : Subsystem
  Encode_RQST : Subsystem
  RQST_13_E4_PGN : Subsystem
  wires:
  Bus Selector/1 -> CAN_TX_RQST_13_E4/2(OperatorEnable)  "<OperatorEnableSwitch>"
  5000msCAN/1 -> Bus Selector/1
  Encode_RQST/1(Data) -> CAN_TX_RQST_13_E4/1(RawData)
  RQST_13_E4_PGN/1(PGN) -> Encode_RQST/1(PGN)

== system SUB_ECU_L4_MABX_HW_Interface_PIC_PB/CAN_Out_PIC_PB/CAN_TX_50ms ==
  50msCAN : Inport
  CAN_TX_CCVS1 : Subsystem
  CAN_TX_TC1_05 : Subsystem
  enable_CAN_TX_CCVS1_CAN3 : Constant  Value=0  OutDataTypeStr=Inherit: Inherit via back propagation
  wires:
  enable_CAN_TX_CCVS1_CAN3/1 -> CAN_TX_CCVS1/2(enable)
  50msCAN/1 -> CAN_TX_CCVS1/1(In1), CAN_TX_TC1_05/1(In1)

== system SUB_ECU_L4_MABX_HW_Interface_PIC_PB/CAN_Out_PIC_PB/CAN_TX_BAM ==
  CM : Subsystem
  Chart : Stateflow chart  TreatAsAtomicUnit=on
  Constant1 : Constant  Value=2  OutDataTypeStr=uint8
  DataFrame1 : Subsystem
  DataFrame2 : Subsystem
  Multiport Switch : MultiPortSwitch  Inputs=2  DiagnosticForDefault=Warning
  TX_TPCM : Subsystem
  TX_TPDT : Subsystem
  Terminator{,1..4} (5 alike) : Terminator
  Unit Delay1 : UnitDelay  InitialCondition=1  SampleTime=-1
  Unit Delay2 : UnitDelay  SampleTime=-1
  Unit Delay3 : UnitDelay  SampleTime=-1
  wires:
  Chart/5(TPDT_ts_Prev) -> Terminator4/1
  Chart/4(TPCM_ts_Prev) -> Terminator3/1
  Unit Delay1/1 -> Multiport Switch/1
  Unit Delay3/1 -> TX_TPDT/1(Trigger)
  Unit Delay2/1 -> TX_TPCM/1(Trigger)
  TX_TPDT/1(TX_status) -> Terminator1/1
  Chart/1(State) -> Terminator/1
  TX_TPCM/1(TX_status) -> Terminator2/1
  Chart/6(TPDT_count) -> Unit Delay1/1
  Chart/3(enTPCM) -> Unit Delay2/1
  Multiport Switch/1 -> TX_TPDT/2(Data)
  Constant1/1 -> Chart/3(TPDT_total)
  CM/1(Out1) -> TX_TPCM/2(Data)
  DataFrame2/1(Out1) -> Multiport Switch/3
  Chart/2(enTPDT) -> Unit Delay3/1
  DataFrame1/1(Out1) -> Multiport Switch/2
  TX_TPCM/2(TX_time) -> Chart/1(TPCM_ts)
  TX_TPDT/2(TX_time) -> Chart/2(TPDT_ts)

== system SUB_ECU_L4_MABX_HW_Interface_PIC_PB/CAN_Out_PIC_PB/CAN_TX_VariableRate ==
  Feedthrough : Inport
  CAN_TX_Std_SystemTime_01 : Subsystem
  wires:
  Feedthrough/1 -> CAN_TX_Std_SystemTime_01/1(Feedthrough)
